simulink model "gm_sampleModel1944_1_sub_sub"  (R2023a)
settings: Solver=VariableStepAuto  StartTime=0.0  StopTime=10.0  RelTol=1e-3
libraries: hdlsllib x2, simulink x1
settings Model: Creator=user1  LastModifiedBy=user1
settings OptimizationCC: BlockReduction=off  ConditionallyExecuteInputs=off
settings DebuggingCC: InheritedTsInSrcMsg=none

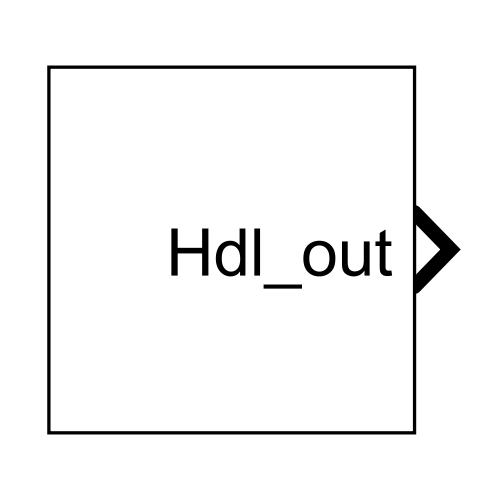
[thumbnail: Simulink's stored preview of the top-level diagram]
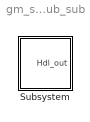
== system gm_sampleModel1944_1_sub_sub ==
  Subsystem : Subsystem

== system gm_sampleModel1944_1_sub_sub/Subsystem ==
  Subsystem : Subsystem
  Hdl_out : Outport  OutDataTypeStr=uint8  SampleTime=1
  wires:
  Subsystem/1(cfblk146) -> Hdl_out/1

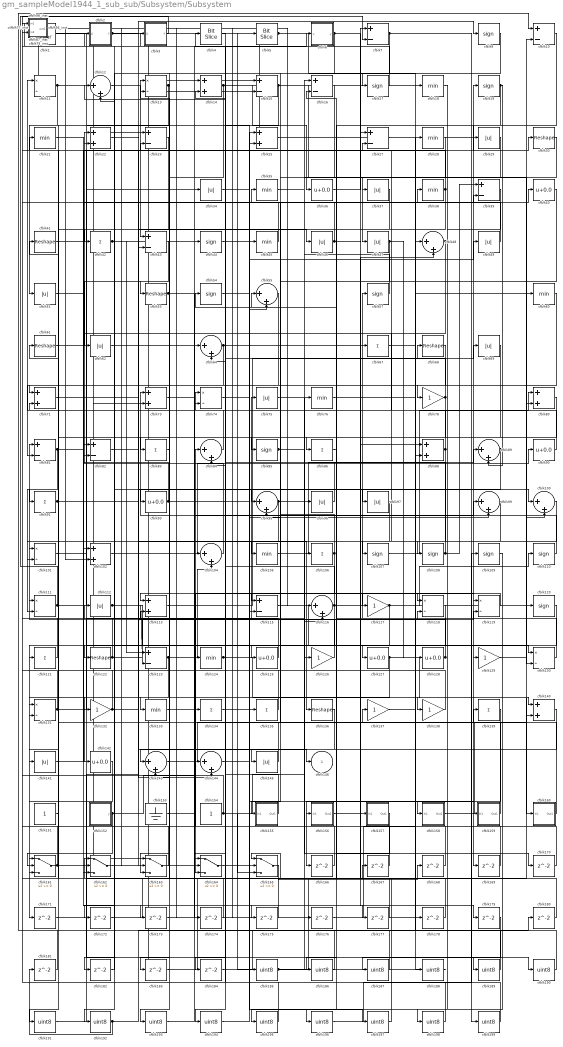
== system gm_sampleModel1944_1_sub_sub/Subsystem/Subsystem ==
  cfblk1 : simulink/Logic and Bit Operations/Bit Clear  iBit=0
      settings: LibrarySourceBlock=|
      | hdlsllib/Logic and Bit
      | Operations/Bit Clear
  cfblk{7,10,15..16,23,27,39,43,81..82,115,123} (12 alike) : Sum  Inputs=+-  OutDataTypeStr=uint8
  cfblk{12,48,55,64,84,89,95,99..100,104,116,143..144} (13 alike) : Sum  Inputs=|++  OutDataTypeStr=uint8
  cfblk{11,13,74,101,111,118..119,130..131} (9 alike) : Product  Inputs=*/  OutDataTypeStr=uint8  RndMeth=Zero  SaturateOnIntegerOverflow=on
  cfblk{14,22,25,71,73,80,88,102,113,140} (10 alike) : Sum  OutDataTypeStr=uint8
  cfblk103_inst : Subsystem
  cfblk{18,21,28,35,38,45,60,76,105,124,133} (11 alike) : MinMax  OutDataTypeStr=uint8
  cfblk{42,67,83,86,91,106,121,134..135,139} (10 alike) : Sum  Inputs=+  OutDataTypeStr=uint8
  cfblk{9,17,19,44,54,57,85,107..110,120} (12 alike) : Signum
  cfblk{29,34,37,46..47,49,51,62,69,75,96..97,112,141,145} (15 alike) : Abs  OutDataTypeStr=uint8  SaturateOnIntegerOverflow=off
  cfblk{78,117,126,129,132,137..138} (7 alike) : Gain  OutDataTypeStr=uint8
  cfblk{30,41,53,61,68,122,136} (7 alike) : Reshape
  cfblk{36,40,90,93,125,127..128,142} (8 alike) : Bias  Bias=0.0  SaturateOnIntegerOverflow=off
  cfblk151 : Constant  OutDataTypeStr=uint8  SampleTime=-1
  cfblk152 : Subsystem  mask(Counter Limited){uplimit=double(7), tsamp=double(-1)}
      mask prompts: uplimit "Simulink:masks:UpperLimit_MP"; tsamp "Simulink:masks:SampleTime_MP"
      mask help: Simulink:masks:CounterLimited_MD
      mask init:
      | nbits = double(8);
      | tsamp = double(-1);
      | uplimit = double(7);
  cfblk153 : Ground
  cfblk154 : Constant  OutDataTypeStr=uint8  SampleTime=-1
  cfblk155 : Subsystem
  cfblk156 : Subsystem
  cfblk157 : Subsystem
  cfblk158 : Subsystem
  cfblk159 : Subsystem
  cfblk160 : Subsystem
  cfblk{161..165} (5 alike) : Switch  OutDataTypeStr=uint8  SaturateOnIntegerOverflow=off  InputSameDT=off
  cfblk{166..184} (19 alike) : Delay  SampleTime=1
  cfblk{185..199} (15 alike) : DataTypeConversion  OutDataTypeStr=uint8  SaturateOnIntegerOverflow=off  RndMeth=Floor
  cfblk2 : Subsystem  mask(Detect Rise Positive){vinit=double(0), InputProcessing=Elements as channels (sample based), OutDataTypeStr=uint8}
      mask prompts: vinit "Simulink:masks:InitialCondition_MP"; InputProcessing "Simulink:masks:InputProcessing_MP"; OutDataTypeStr "Simulink:masks:OutputDataType_MP"
      mask help: Simulink:masks:DetectRisePositive_MD
      mask init:
      | InputProcessing = 'Elements as channels (sample based)';
      | OutDataTypeStr = 'uint8';
      | vinit = double(0);
      mask TypeOptions InputProcessing: Simulink:masks:ColumnsAsChannelsFrameBased | Simulink:masks:ElementsAsChannelsSampleBased
      mask TypeOptions OutDataTypeStr: Simulink:masks:uint8 | Simulink:masks:boolean
      mask Display: fprintf('U > 0\n&  NOT\nU/z > 0')
  cfblk3 : Subsystem  mask(Detect Fall Nonpositive){vinit=double(0), InputProcessing=Elements as channels (sample based), OutDataTypeStr=uint8}
      mask prompts: vinit "Simulink:masks:InitialCondition_MP"; InputProcessing "Simulink:masks:InputProcessing_MP"; OutDataTypeStr "Simulink:masks:OutputDataType_MP"
      mask help: Simulink:masks:DetectFallNonpositive_MD
      mask init:
      | InputProcessing = 'Elements as channels (sample based)';
      | OutDataTypeStr = 'uint8';
      | vinit = double(0);
      mask TypeOptions InputProcessing: Simulink:masks:ColumnsAsChannelsFrameBased | Simulink:masks:ElementsAsChannelsSampleBased
      mask TypeOptions OutDataTypeStr: Simulink:masks:uint8 | Simulink:masks:boolean
      mask Display: fprintf('U <= 0\n&  NOT\nU/z <= 0')
  cfblk32_inst : Subsystem
  cfblk33_inst : Subsystem
  cfblk4 : hdlsllib/Logic and Bit Operations/Bit Slice  lidx=7  ridx=0
  cfblk5 : hdlsllib/Logic and Bit Operations/Bit Slice  lidx=7  ridx=0
  cfblk52_inst : Subsystem
  cfblk6 : Subsystem  mask(Compare To Constant){relop=<=, const=double(3), OutDataTypeStr=uint8, ZeroCross=on}
      mask prompts: relop "Simulink:masks:Operator_MP"; const "Simulink:masks:ConstantValue_MP"; OutDataTypeStr "Simulink:masks:OutputDataType_MP"; ZeroCross "Simulink:masks:EnableZerocrossingDetection_MP"
      mask help: Simulink:masks:CompareToConstant_MD
      mask init:
      | OutDataTypeStr = 'uint8';
      | ZeroCross = 'on';
      | blkName = 'sampleModel1944_1_sub_sub/Subsystem/Subsystem/cfblk6';
      | const = double(3);
      | const_str = '3.0';
      | const_val = double(3);
      | relop = '<=';
      | setValue = 'fixdt(0, 8)';
      | str = '<= 3';
      mask TypeOptions relop: == | ~= | < | <= | >= | >
      mask TypeOptions OutDataTypeStr: Simulink:masks:uint8 | Simulink:masks:boolean
      mask Callback ZeroCross: sl('zeroCrossEnable', gcbh);
      mask Display: disp(str)
  cfblk66_inst : Subsystem
  cfblk70_inst : Subsystem
  cfblk77_inst : Subsystem
  cfblk79_inst : Subsystem
  cfblk87_inst : Subsystem
  cfblk94_inst : Subsystem
  cfblk98_inst : Subsystem
  cfblk146 : Outport  OutDataTypeStr=uint8  SampleTime=1  VectorParamsAs1DForOutWhenUnconnected=off
  wires:
  cfblk1/1 -> cfblk189/1
  cfblk10/1 -> cfblk169/1
  cfblk100/1 -> cfblk136/1
  cfblk101/1 -> cfblk127/1
  cfblk102/1 -> cfblk90/1
  cfblk103_inst/1(out1) -> cfblk11/2, cfblk18/1
  cfblk104/1 -> cfblk22/1
  cfblk105/1 -> cfblk89/1
  cfblk106/1 -> cfblk55/1, cfblk164/3
  cfblk107/1 -> cfblk80/1
  cfblk108/1 -> cfblk98_inst/1(in1), cfblk39/1
  cfblk109/1 -> cfblk195/1
  cfblk11/1 -> cfblk51/1, cfblk135/1
  cfblk110/1 -> cfblk73/1
  cfblk111/1 -> cfblk7/2, cfblk34/1
  cfblk112/1 -> cfblk123/2, cfblk157/1(In1)
  cfblk113/1 -> cfblk69/1
  cfblk115/1 -> cfblk130/1
  cfblk116/1 -> cfblk32_inst/2(in2), cfblk113/1, cfblk171/1
  cfblk117/1 -> cfblk161/3, cfblk110/1
  cfblk118/1 -> cfblk193/1
  cfblk119/1 -> cfblk116/1
  cfblk12/1 -> cfblk43/1
  cfblk120/1 -> cfblk133/1
  cfblk121/1 -> cfblk70_inst/2(in2)
  cfblk122/1 -> cfblk79_inst/2(in2), cfblk39/2, cfblk103_inst/2(in2)
  cfblk123/1 -> cfblk104/2, cfblk131/2
  cfblk124/1 -> cfblk140/1, cfblk160/1(In1)
  cfblk125/1 -> cfblk81/1
  cfblk126/1 -> cfblk112/1
  cfblk127/1 -> cfblk194/1, cfblk142/1, cfblk140/2
  cfblk128/1 -> cfblk54/1, cfblk111/1
  cfblk129/1 -> cfblk10/2
  cfblk13/1 -> cfblk141/1, cfblk83/1
  cfblk130/1 -> cfblk57/1
  cfblk131/1 -> cfblk79_inst/1(in1), cfblk75/1, cfblk68/1, cfblk25/2
  cfblk132/1 -> cfblk61/1, cfblk118/2
  cfblk133/1 -> cfblk84/1
  cfblk134/1 -> cfblk55/2
  cfblk135/1 -> cfblk14/2
  cfblk136/1 -> cfblk145/1
  cfblk137/1 -> cfblk28/1
  cfblk138/1 -> cfblk101/1
  cfblk139/1 -> cfblk166/1
  cfblk14/1 -> cfblk36/1, cfblk163/3
  cfblk140/1 -> cfblk143/1
  cfblk141/1 -> cfblk82/1
  cfblk142/1 -> cfblk161/1
  cfblk143/1 -> cfblk139/1
  cfblk144/1 -> cfblk137/1
  cfblk145/1 -> cfblk21/1
  cfblk15/1 -> cfblk130/2, cfblk124/1
  cfblk151/1 -> cfblk10/1
  cfblk152/1(y) -> cfblk161/2, cfblk134/1
  cfblk153/1 -> cfblk64/1
  cfblk154/1 -> cfblk96/1, cfblk52_inst/1(in1), cfblk165/3, cfblk113/2
  cfblk155/1(Out1) -> cfblk12/1
  cfblk156/1(Out1) -> cfblk48/2
  cfblk157/1(Out1) -> cfblk165/1
  cfblk158/1(Out1) -> cfblk100/2
  cfblk159/1(Out1) -> cfblk35/1
  cfblk16/1 -> cfblk85/1
  cfblk160/1(Out1) -> cfblk41/1
  cfblk161/1 -> cfblk52_inst/2(in2), cfblk175/1
  cfblk162/1 -> cfblk43/2
  cfblk163/1 -> cfblk82/2
  cfblk164/1 -> cfblk165/2
  cfblk165/1 -> cfblk168/1
  cfblk166/1 -> cfblk13/1
  cfblk167/1 -> cfblk87_inst/1(in1)
  cfblk168/1 -> cfblk70_inst/1(in1)
  cfblk169/1 -> cfblk144/1
  cfblk17/1 -> cfblk3/1(U)
  cfblk170/1 -> cfblk2/1(U)
  cfblk171/1 -> cfblk119/2
  cfblk172/1 -> cfblk116/2
  cfblk173/1 -> cfblk80/2
  cfblk174/1 -> cfblk66_inst/2(in2)
  cfblk175/1 -> cfblk162/1
  cfblk176/1 -> cfblk48/1
  cfblk177/1 -> cfblk71/2
  cfblk178/1 -> cfblk23/2
  cfblk179/1 -> cfblk187/1
  cfblk18/1 -> cfblk78/1
  cfblk180/1 -> cfblk16/2
  cfblk181/1 -> cfblk94_inst/2(in2)
  cfblk182/1 -> cfblk22/2
  cfblk183/1 -> cfblk115/2
  cfblk184/1 -> cfblk88/2
  cfblk185/1 -> cfblk126/1, cfblk67/1
  cfblk186/1 -> cfblk33_inst/1(in1)
  cfblk187/1 -> cfblk33_inst/2(in2)
  cfblk188/1 -> cfblk1/1
  cfblk189/1 -> cfblk77_inst/1(in1)
  cfblk19/1 -> cfblk89/2, cfblk186/1
  cfblk190/1 -> cfblk77_inst/2(in2)
  cfblk191/1 -> cfblk76/1
  cfblk192/1 -> cfblk181/1, cfblk180/1
  cfblk193/1 -> cfblk99/1
  cfblk194/1 -> cfblk99/2
  cfblk195/1 -> cfblk87_inst/2(in2)
  cfblk196/1 -> cfblk109/1
  cfblk197/1 -> cfblk167/1
  cfblk198/1 -> cfblk74/1
  cfblk199/1 -> cfblk74/2
  cfblk2/1(Y) -> cfblk9/1, cfblk106/1
  cfblk21/1 -> cfblk173/1
  cfblk22/1 -> cfblk46/1
  cfblk23/1 -> cfblk71/1
  cfblk25/1 -> cfblk7/1
  cfblk27/1 -> cfblk129/1
  cfblk28/1 -> cfblk86/1
  cfblk29/1 -> cfblk105/1
  cfblk3/1(Y) -> cfblk94_inst/1(in1)
  cfblk30/1 -> cfblk47/1
  cfblk32_inst/1(out1) -> cfblk178/1
  cfblk33_inst/1(out1) -> cfblk185/1
  cfblk34/1 -> cfblk159/1(In1)
  cfblk35/1 -> cfblk37/1
  cfblk36/1 -> cfblk27/1
  cfblk37/1 -> cfblk122/1
  cfblk38/1 -> cfblk32_inst/1(in1), cfblk182/1, cfblk91/1
  cfblk39/1 -> cfblk198/1
  cfblk4/1 -> cfblk84/2
  cfblk40/1 -> cfblk155/1(In1)
  cfblk41/1 -> cfblk19/1
  cfblk42/1 -> cfblk125/1, cfblk123/1, cfblk104/1
  cfblk43/1 -> cfblk62/1
  cfblk44/1 -> cfblk64/2
  cfblk45/1 -> cfblk13/2
  cfblk46/1 -> cfblk98_inst/2(in2), cfblk88/1
  cfblk47/1 -> cfblk196/1, cfblk128/1
  cfblk48/1 -> cfblk162/2, cfblk107/1
  cfblk49/1 -> cfblk66_inst/1(in1)
  cfblk5/1 -> cfblk188/1, cfblk17/1
  cfblk51/1 -> cfblk102/1
  cfblk52_inst/1(out1) -> cfblk73/2, cfblk176/1
  cfblk53/1 -> cfblk119/1, cfblk6/1(u)
  cfblk54/1 -> cfblk158/1(In1)
  cfblk55/1 -> cfblk132/1
  cfblk57/1 -> cfblk16/1
  cfblk6/1(y) -> cfblk95/1, cfblk179/1
  cfblk60/1 -> cfblk108/1
  cfblk61/1 -> cfblk30/1
  cfblk62/1 -> cfblk117/1
  cfblk64/1 -> cfblk81/2, cfblk5/1, cfblk163/2, cfblk138/1
  cfblk66_inst/1(out1) -> cfblk29/1, cfblk164/2
  cfblk67/1 -> cfblk60/1
  cfblk68/1 -> cfblk191/1
  cfblk69/1 -> cfblk93/1
  cfblk7/1 -> cfblk53/1, cfblk199/1, cfblk164/1
  cfblk70_inst/1(out1) -> cfblk44/1
  cfblk71/1 -> cfblk144/2
  cfblk73/1 -> cfblk174/1
  cfblk74/1 -> cfblk197/1
  cfblk75/1 -> cfblk170/1
  cfblk76/1 -> cfblk190/1
  cfblk77_inst/1(out1) -> cfblk45/1
  cfblk78/1 -> cfblk4/1, cfblk184/1, cfblk183/1
  cfblk79_inst/1(out1) -> cfblk120/1
  cfblk80/1 -> cfblk121/1
  cfblk81/1 -> cfblk40/1, cfblk101/2
  cfblk82/1 -> cfblk146/1
  cfblk83/1 -> cfblk143/2
  cfblk84/1 -> cfblk11/1
  cfblk85/1 -> cfblk118/1, cfblk38/1
  cfblk86/1 -> cfblk156/1(In1)
  cfblk87_inst/1(out1) -> cfblk23/1
  cfblk88/1 -> cfblk27/2, cfblk115/1, cfblk131/1
  cfblk89/1 -> cfblk95/2, cfblk172/1
  cfblk9/1 -> cfblk42/1
  cfblk90/1 -> cfblk14/1
  cfblk91/1 -> cfblk97/1, cfblk25/1
  cfblk93/1 -> cfblk49/1, cfblk12/2, cfblk177/1
  cfblk94_inst/1(out1) -> cfblk15/2, cfblk15/1, cfblk102/2
  cfblk95/1 -> cfblk162/3, cfblk100/1
  cfblk96/1 -> cfblk103_inst/1(in1)
  cfblk97/1 -> cfblk111/2
  cfblk98_inst/1(out1) -> cfblk163/1
  cfblk99/1 -> cfblk192/1

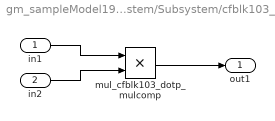
== system gm_sampleModel1944_1_sub_sub/Subsystem/Subsystem/cfblk103_inst ==
  in1 : Inport  OutDataTypeStr=uint8  SampleTime=1
  in2 : Inport  Port=2  OutDataTypeStr=uint8  SampleTime=1
  mul_cfblk103_dotp_mulcomp : Product  Inputs=**  OutDataTypeStr=uint8  SampleTime=1
  out1 : Outport  OutDataTypeStr=uint8  SampleTime=1
  wires:
  in1/1 -> mul_cfblk103_dotp_mulcomp/1
  in2/1 -> mul_cfblk103_dotp_mulcomp/2
  mul_cfblk103_dotp_mulcomp/1 -> out1/1

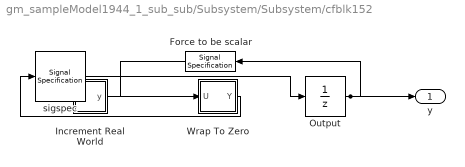
== system gm_sampleModel1944_1_sub_sub/Subsystem/Subsystem/cfblk152 ==
  Force to be scalar : SignalSpecification  DisableCoverage=on  Dimensions=1
  Increment Real World : Subsystem  mask(Real World Value Increment){}
      mask help: Simulink:masks:RealWorldValueIncrement_MD
      mask Display: disp('V++')
  Output : UnitDelay  InitialCondition=0.0  SampleTime=tsamp  HasFrameUpgradeWarning=on
  Wrap To Zero : Subsystem  mask(Wrap To Zero){Threshold=double(7)}
      mask prompts: Threshold "Simulink:masks:Threshold_MP"
      mask help: Simulink:masks:WrapToZero_MD
  sigspec : SignalSpecification  OutDataTypeStr=uint8  Dimensions=1
  y : Outport  SampleTime=1
  wires:
  Force to be scalar/1 -> Increment Real World/1(u)
  Increment Real World/1(y) -> Wrap To Zero/1(U)
  Output/1 -> Force to be scalar/1, y/1
  Wrap To Zero/1(Y) -> sigspec/1
  sigspec/1 -> Output/1

== system gm_sampleModel1944_1_sub_sub/Subsystem/Subsystem/cfblk155 ==
  In1 : Inport  OutDataTypeStr=uint8  PortDimensions=1  SampleTime=1
  Out1 : Outport  SampleTime=1
  wires:
  In1/1 -> Out1/1

== system gm_sampleModel1944_1_sub_sub/Subsystem/Subsystem/cfblk156 ==
  In1 : Inport  OutDataTypeStr=uint8  PortDimensions=1  SampleTime=1
  Out1 : Outport  SampleTime=1
  wires:
  In1/1 -> Out1/1

== system gm_sampleModel1944_1_sub_sub/Subsystem/Subsystem/cfblk157 ==
  In1 : Inport  OutDataTypeStr=uint8  PortDimensions=1  SampleTime=1
  Out1 : Outport  SampleTime=1
  wires:
  In1/1 -> Out1/1

== system gm_sampleModel1944_1_sub_sub/Subsystem/Subsystem/cfblk158 ==
  In1 : Inport  OutDataTypeStr=uint8  PortDimensions=1  SampleTime=1
  Out1 : Outport  SampleTime=1
  wires:
  In1/1 -> Out1/1

== system gm_sampleModel1944_1_sub_sub/Subsystem/Subsystem/cfblk159 ==
  In1 : Inport  OutDataTypeStr=uint8  PortDimensions=1  SampleTime=1
  Out1 : Outport  SampleTime=1
  wires:
  In1/1 -> Out1/1

== system gm_sampleModel1944_1_sub_sub/Subsystem/Subsystem/cfblk160 ==
  In1 : Inport  OutDataTypeStr=uint8  PortDimensions=1  SampleTime=1
  Out1 : Outport  SampleTime=1
  wires:
  In1/1 -> Out1/1

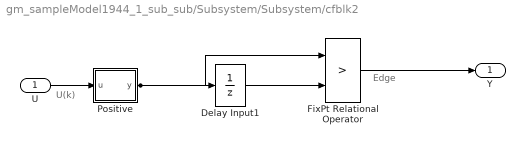
== system gm_sampleModel1944_1_sub_sub/Subsystem/Subsystem/cfblk2 ==
  note: U(k)
  note: Edge
  U : Inport  OutDataTypeStr=uint8  SampleTime=1
  Delay Input1 : UnitDelay  Description=Store in Global RAM  DisableCoverage=on  InitialCondition=vinit  SampleTime=-1  HasFrameUpgradeWarning=on
  FixPt Relational Operator : RelationalOperator  Operator=>  OutDataTypeStr=fixdt(0, 8)  ZeroCross=off  InputSameDT=off
  Positive : Subsystem  mask(Compare To Zero){relop=>, OutDataTypeStr=boolean, ZeroCross=off}
      mask prompts: relop "Simulink:masks:Operator_MP"; OutDataTypeStr "Simulink:masks:OutputDataType_MP"; ZeroCross "Simulink:masks:EnableZerocrossingDetection_MP"
      mask help: Simulink:masks:CompareToZero_MD
      mask init:
      | OutDataTypeStr = 'boolean';
      | ZeroCross = 'off';
      | blkName = 'sampleModel1944_1_sub_sub/Subsystem/Subsystem/cfblk2/Positive';
      | relop = '>';
      | setValue = 'boolean';
      mask TypeOptions relop: == | ~= | < | <= | >= | >
      mask TypeOptions OutDataTypeStr: Simulink:masks:uint8 | Simulink:masks:boolean
      mask Callback ZeroCross: sl('zeroCrossEnable', gcbh);
      mask Display: disp([relop,' 0'])
  Y : Outport  SampleTime=1
  wires:
  U/1 -> Positive/1(u)
  Delay Input1/1 -> FixPt Relational Operator/2
  FixPt Relational Operator/1 -> Y/1
  Positive/1(y) -> FixPt Relational Operator/1, Delay Input1/1

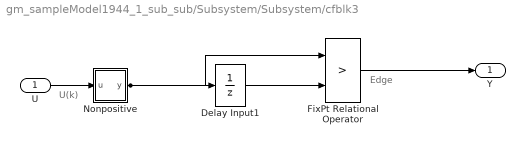
== system gm_sampleModel1944_1_sub_sub/Subsystem/Subsystem/cfblk3 ==
  note: U(k)
  note: Edge
  U : Inport  OutDataTypeStr=uint8  SampleTime=1
  Delay Input1 : UnitDelay  Description=Store in Global RAM  DisableCoverage=on  InitialCondition=vinit  SampleTime=-1  HasFrameUpgradeWarning=on
  FixPt Relational Operator : RelationalOperator  Operator=>  OutDataTypeStr=fixdt(0, 8)  ZeroCross=off  InputSameDT=off
  Nonpositive : Subsystem  mask(Compare To Zero){relop=<=, OutDataTypeStr=boolean, ZeroCross=off}
      mask prompts: relop "Simulink:masks:Operator_MP"; OutDataTypeStr "Simulink:masks:OutputDataType_MP"; ZeroCross "Simulink:masks:EnableZerocrossingDetection_MP"
      mask help: Simulink:masks:CompareToZero_MD
      mask init:
      | OutDataTypeStr = 'boolean';
      | ZeroCross = 'off';
      | blkName = 'sampleModel1944_1_sub_sub/Subsystem/Subsystem/cfblk3/Nonpositive';
      | relop = '<=';
      | setValue = 'boolean';
      mask TypeOptions relop: == | ~= | < | <= | >= | >
      mask TypeOptions OutDataTypeStr: Simulink:masks:uint8 | Simulink:masks:boolean
      mask Callback ZeroCross: sl('zeroCrossEnable', gcbh);
      mask Display: disp([relop,' 0'])
  Y : Outport  SampleTime=1
  wires:
  U/1 -> Nonpositive/1(u)
  Delay Input1/1 -> FixPt Relational Operator/2
  FixPt Relational Operator/1 -> Y/1
  Nonpositive/1(y) -> FixPt Relational Operator/1, Delay Input1/1

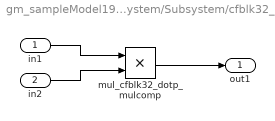
== system gm_sampleModel1944_1_sub_sub/Subsystem/Subsystem/cfblk32_inst ==
  in1 : Inport  OutDataTypeStr=uint8  SampleTime=1
  in2 : Inport  Port=2  OutDataTypeStr=uint8  SampleTime=1
  mul_cfblk32_dotp_mulcomp : Product  Inputs=**  OutDataTypeStr=uint8  SampleTime=1
  out1 : Outport  OutDataTypeStr=uint8  SampleTime=1
  wires:
  in1/1 -> mul_cfblk32_dotp_mulcomp/1
  in2/1 -> mul_cfblk32_dotp_mulcomp/2
  mul_cfblk32_dotp_mulcomp/1 -> out1/1

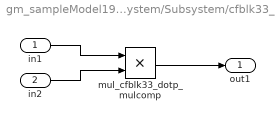
== system gm_sampleModel1944_1_sub_sub/Subsystem/Subsystem/cfblk33_inst ==
  in1 : Inport  OutDataTypeStr=uint8  SampleTime=1
  in2 : Inport  Port=2  OutDataTypeStr=uint8  SampleTime=1
  mul_cfblk33_dotp_mulcomp : Product  Inputs=**  OutDataTypeStr=uint8  SampleTime=1
  out1 : Outport  OutDataTypeStr=uint8  SampleTime=1
  wires:
  in1/1 -> mul_cfblk33_dotp_mulcomp/1
  in2/1 -> mul_cfblk33_dotp_mulcomp/2
  mul_cfblk33_dotp_mulcomp/1 -> out1/1

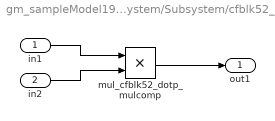
== system gm_sampleModel1944_1_sub_sub/Subsystem/Subsystem/cfblk52_inst ==
  in1 : Inport  OutDataTypeStr=uint8  SampleTime=1
  in2 : Inport  Port=2  OutDataTypeStr=uint8  SampleTime=1
  mul_cfblk52_dotp_mulcomp : Product  Inputs=**  OutDataTypeStr=uint8  SampleTime=1
  out1 : Outport  OutDataTypeStr=uint8  SampleTime=1
  wires:
  in1/1 -> mul_cfblk52_dotp_mulcomp/1
  in2/1 -> mul_cfblk52_dotp_mulcomp/2
  mul_cfblk52_dotp_mulcomp/1 -> out1/1

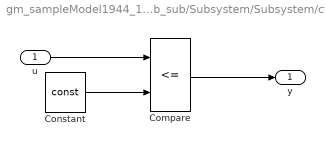
== system gm_sampleModel1944_1_sub_sub/Subsystem/Subsystem/cfblk6 ==
  u : Inport  OutDataTypeStr=uint8  SampleTime=1
  Compare : RelationalOperator  Operator=<=  OutDataTypeStr=fixdt(0, 8)
  Constant : Constant  DisableCoverage=on  Value=const  OutDataTypeStr=Inherit: Inherit via back propagation  SampleTime=-1
  y : Outport  SampleTime=1
  wires:
  u/1 -> Compare/1
  Compare/1 -> y/1
  Constant/1 -> Compare/2

== system gm_sampleModel1944_1_sub_sub/Subsystem/Subsystem/cfblk66_inst ==
  in1 : Inport  OutDataTypeStr=uint8  SampleTime=1
  in2 : Inport  Port=2  OutDataTypeStr=uint8  SampleTime=1
  mul_cfblk66_dotp_mulcomp : Product  Inputs=**  OutDataTypeStr=uint8  SampleTime=1
  out1 : Outport  OutDataTypeStr=uint8  SampleTime=1
  wires:
  in1/1 -> mul_cfblk66_dotp_mulcomp/1
  in2/1 -> mul_cfblk66_dotp_mulcomp/2
  mul_cfblk66_dotp_mulcomp/1 -> out1/1

== system gm_sampleModel1944_1_sub_sub/Subsystem/Subsystem/cfblk70_inst ==
  in1 : Inport  OutDataTypeStr=uint8  SampleTime=1
  in2 : Inport  Port=2  OutDataTypeStr=uint8  SampleTime=1
  mul_cfblk70_dotp_mulcomp : Product  Inputs=**  OutDataTypeStr=uint8  SampleTime=1
  out1 : Outport  OutDataTypeStr=uint8  SampleTime=1
  wires:
  in1/1 -> mul_cfblk70_dotp_mulcomp/1
  in2/1 -> mul_cfblk70_dotp_mulcomp/2
  mul_cfblk70_dotp_mulcomp/1 -> out1/1

== system gm_sampleModel1944_1_sub_sub/Subsystem/Subsystem/cfblk77_inst ==
  in1 : Inport  OutDataTypeStr=uint8  SampleTime=1
  in2 : Inport  Port=2  OutDataTypeStr=uint8  SampleTime=1
  mul_cfblk77_dotp_mulcomp : Product  Inputs=**  OutDataTypeStr=uint8  SampleTime=1
  out1 : Outport  OutDataTypeStr=uint8  SampleTime=1
  wires:
  in1/1 -> mul_cfblk77_dotp_mulcomp/1
  in2/1 -> mul_cfblk77_dotp_mulcomp/2
  mul_cfblk77_dotp_mulcomp/1 -> out1/1

== system gm_sampleModel1944_1_sub_sub/Subsystem/Subsystem/cfblk79_inst ==
  in1 : Inport  OutDataTypeStr=uint8  SampleTime=1
  in2 : Inport  Port=2  OutDataTypeStr=uint8  SampleTime=1
  mul_cfblk79_dotp_mulcomp : Product  Inputs=**  OutDataTypeStr=uint8  SampleTime=1
  out1 : Outport  OutDataTypeStr=uint8  SampleTime=1
  wires:
  in1/1 -> mul_cfblk79_dotp_mulcomp/1
  in2/1 -> mul_cfblk79_dotp_mulcomp/2
  mul_cfblk79_dotp_mulcomp/1 -> out1/1

== system gm_sampleModel1944_1_sub_sub/Subsystem/Subsystem/cfblk87_inst ==
  in1 : Inport  OutDataTypeStr=uint8  SampleTime=1
  in2 : Inport  Port=2  OutDataTypeStr=uint8  SampleTime=1
  mul_cfblk87_dotp_mulcomp : Product  Inputs=**  OutDataTypeStr=uint8  SampleTime=1
  out1 : Outport  OutDataTypeStr=uint8  SampleTime=1
  wires:
  in1/1 -> mul_cfblk87_dotp_mulcomp/1
  in2/1 -> mul_cfblk87_dotp_mulcomp/2
  mul_cfblk87_dotp_mulcomp/1 -> out1/1

== system gm_sampleModel1944_1_sub_sub/Subsystem/Subsystem/cfblk94_inst ==
  in1 : Inport  OutDataTypeStr=uint8  SampleTime=1
  in2 : Inport  Port=2  OutDataTypeStr=uint8  SampleTime=1
  mul_cfblk94_dotp_mulcomp : Product  Inputs=**  OutDataTypeStr=uint8  SampleTime=1
  out1 : Outport  OutDataTypeStr=uint8  SampleTime=1
  wires:
  in1/1 -> mul_cfblk94_dotp_mulcomp/1
  in2/1 -> mul_cfblk94_dotp_mulcomp/2
  mul_cfblk94_dotp_mulcomp/1 -> out1/1

== system gm_sampleModel1944_1_sub_sub/Subsystem/Subsystem/cfblk98_inst ==
  in1 : Inport  OutDataTypeStr=uint8  SampleTime=1
  in2 : Inport  Port=2  OutDataTypeStr=uint8  SampleTime=1
  mul_cfblk98_dotp_mulcomp : Product  Inputs=**  OutDataTypeStr=uint8  SampleTime=1
  out1 : Outport  OutDataTypeStr=uint8  SampleTime=1
  wires:
  in1/1 -> mul_cfblk98_dotp_mulcomp/1
  in2/1 -> mul_cfblk98_dotp_mulcomp/2
  mul_cfblk98_dotp_mulcomp/1 -> out1/1

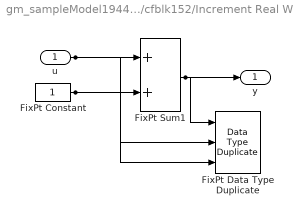
== system gm_sampleModel1944_1_sub_sub/Subsystem/Subsystem/cfblk152/Increment Real World ==
  u : Inport  OutDataTypeStr=uint8  SampleTime=1
  FixPt Constant : Constant  DisableCoverage=on  OutDataTypeStr=Inherit: Inherit via back propagation  SampleTime=-1
  FixPt Data Type Duplicate : DataTypeDuplicate  DisableCoverage=on  NumInputPorts=3
  FixPt Sum1 : Sum  InputSameDT=on  OutDataTypeStr=Inherit: Inherit via back propagation  LockScale=on
  y : Outport  SampleTime=1
  wires:
  u/1 -> FixPt Sum1/1, FixPt Data Type Duplicate/2
  FixPt Constant/1 -> FixPt Sum1/2, FixPt Data Type Duplicate/3
  FixPt Sum1/1 -> FixPt Data Type Duplicate/1, y/1

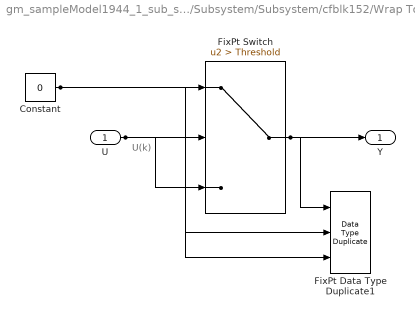
== system gm_sampleModel1944_1_sub_sub/Subsystem/Subsystem/cfblk152/Wrap To Zero ==
  note: U(k)
  U : Inport  OutDataTypeStr=uint8  SampleTime=1
  Constant : Constant  DisableCoverage=on  Value=0  OutDataTypeStr=Inherit: Inherit via back propagation  SampleTime=-1
  FixPt Data Type Duplicate1 : DataTypeDuplicate  DisableCoverage=on  NumInputPorts=3
  FixPt Switch : Switch  Criteria=u2 > Threshold  Threshold=Threshold  OutDataTypeStr=Inherit: Inherit via back propagation  ZeroCross=off  SaturateOnIntegerOverflow=off  InputSameDT=off
  Y : Outport  SampleTime=1
  wires:
  U/1 -> FixPt Switch/3, FixPt Switch/2, FixPt Data Type Duplicate1/2
  Constant/1 -> FixPt Switch/1, FixPt Data Type Duplicate1/3
  FixPt Switch/1 -> FixPt Data Type Duplicate1/1, Y/1

== system gm_sampleModel1944_1_sub_sub/Subsystem/Subsystem/cfblk2/Positive ==
  u : Inport  OutDataTypeStr=uint8  SampleTime=1
  Compare : RelationalOperator  Operator=>  OutDataTypeStr=boolean  ZeroCross=off
  Constant : Constant  DisableCoverage=on  Value=0  OutDataTypeStr=Inherit: Inherit via back propagation  SampleTime=-1  PreserveConstantTs=on
  y : Outport  SampleTime=1
  wires:
  u/1 -> Compare/1
  Compare/1 -> y/1
  Constant/1 -> Compare/2

== system gm_sampleModel1944_1_sub_sub/Subsystem/Subsystem/cfblk3/Nonpositive ==
  u : Inport  OutDataTypeStr=uint8  SampleTime=1
  Compare : RelationalOperator  Operator=<=  OutDataTypeStr=boolean  ZeroCross=off
  Constant : Constant  DisableCoverage=on  Value=0  OutDataTypeStr=Inherit: Inherit via back propagation  SampleTime=-1  PreserveConstantTs=on
  y : Outport  SampleTime=1
  wires:
  u/1 -> Compare/1
  Compare/1 -> y/1
  Constant/1 -> Compare/2
